simulink model "dq_model"  (R2015a)
settings: Solver=ode45  StartTime=0.0  StopTime=1.5  FixedStep=1e-5  MaxStep=1e-3  RelTol=1e-3
InitFcn:
  | parametriAM
values from neighbouring files (symbols this model uses):
  Imrn = 7.4    [parametriAM.m]
  Ismax = In*sqrt(2)    [parametriAM.m]
  J = 0.019    [parametriAM.m]    (also in podatki.m = 0.01)
  Ki_Imr = 1000    [parametriAM.m]
  Ki_tok = 5.0    (= 5)    [parametriAM.m]
  Ki_wr = 1000    [parametriAM.m]
  Kp_Imr = 100    [parametriAM.m]
  Kp_tok = 0.05    [parametriAM.m]
  Kp_wr = 50    [parametriAM.m]
  Lm = 0.0493    [parametriAM.m]    (also in podatki.m = 0.2342)
  Lr = 0.05315    [parametriAM.m]    (also in podatki.m = 0.2449)
  Ls = 0.05315    [parametriAM.m]    (also in podatki.m = 0.2449)
  Lst = sigma*Ls    (= 0.00742111947319)    [parametriAM.m]
  pp = 3    [parametriAM.m]    (also in podatki.m = 2)
  Rs = 0.594    [parametriAM.m]    (also in podatki.m = 3.7)
  sigma = 1 - 1/((1+sigmaR)*(1+sigmaS))    (= 0.13962595434)    [parametriAM.m]
  Tr = Lr/Rr    (= 0.0771407837446)    [parametriAM.m]
  Udc = Un*sqrt(2)    [parametriAM.m]
  wb_upper_limit_field_weaking = sqrt((Ls^2+Lst^2)/(2*Lst^2*Ls^2))*Usmax/Ismax    [parametriAM.m]
  wn = Udc/sqrt(Ls^2*(Imrn)^2+Lst^2*(Ismax^2-(Imrn)^2))    [maximalnaelipsa.m]    (also in parametriAM.m = Un/sqrt(Ls^2*(Imrn)^2+Lst^2*(Ismax^2-(Imrn)^2))/pp)
libraries: simulink x20
(part 1 of 2)
settings Model: CovModelRefEnable=off  Creator=Mitja1  LastModifiedBy=Jan
settings DataIOCC: LimitDataPoints=off  SaveFormat=Dataset
settings HardwareCC: ProdBitPerPointer=64  ProdLargestAtomicFloat=Float  ProdIntDivRoundTo=Zero  ProdEndianess=LittleEndian  ProdHWDeviceType=Specified
settings ModelReferenceCC: PropagateSignalLabelsOutOfModel=on

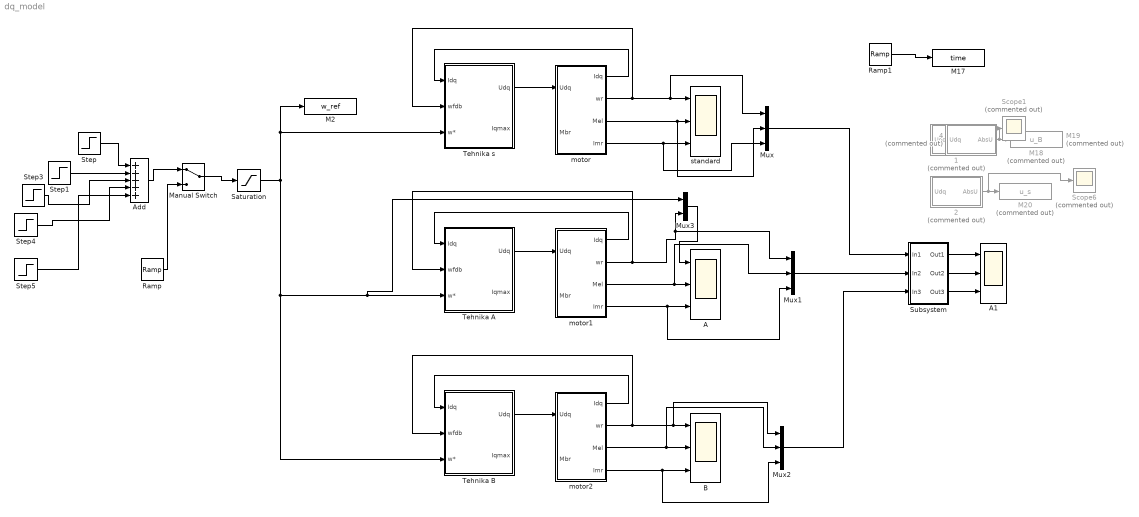
== system dq_model ==
  1 : Subsystem  Commented=on
  2 : Subsystem  Commented=on
  4 : Subsystem  Commented=on
  A : Scope  NumInputPorts=3
      settings: TimeRange=auto  MaxDataPoints=5000  SaveToWorkspace=off  SaveName=ScopeData5  YMin=-48.75~-0.06733~-3.30469  YMax=438.75~0.60598~29.7522  SampleTime=-1
  A1 : Scope  NumInputPorts=3
      settings: TimeRange=auto  MaxDataPoints=5000  SaveToWorkspace=off  SaveName=ScopeData7  YMin=-65.4584~-0.02651~-3.33779  YMax=589.12557~0.12258~30.05009  SampleTime=-1
  Add : Sum  Inputs=+++++
  B : Scope  NumInputPorts=3
      settings: TimeRange=auto  MaxDataPoints=5000  SaveToWorkspace=off  SaveName=ScopeData6  YMin=-28.02182~-2.20302~-3.30355  YMax=252.1964~2.96621~29.74192  SampleTime=-1
  M17 : ToWorkspace  VariableName=time  SampleTime=-1
      settings: Decimation=3  Save2DSignal=2-D array (concatenate along first dimension)
  M18 : ToWorkspace  Commented=on  VariableName=u_A  SampleTime=-1
      settings: Decimation=3  Save2DSignal=2-D array (concatenate along first dimension)
  M19 : ToWorkspace  Commented=on  VariableName=u_B  SampleTime=-1
      settings: Decimation=3  Save2DSignal=2-D array (concatenate along first dimension)
  M2 : ToWorkspace  VariableName=w_ref  SampleTime=-1
      settings: Decimation=3  Save2DSignal=2-D array (concatenate along first dimension)
  M20 : ToWorkspace  Commented=on  VariableName=u_s  SampleTime=-1
      settings: Decimation=3  Save2DSignal=2-D array (concatenate along first dimension)
  Manual Switch : ManualSwitch
  Mux : Mux  Inputs=3
  Mux1 : Mux  Inputs=3
  Mux2 : Mux  Inputs=3
  Mux3 : Mux  Inputs=2
  Ramp : simulink/Sources/Ramp  slope=20  start=0.5  X0=0
  Ramp1 : simulink/Sources/Ramp  slope=1  start=0  X0=0
  Saturation : Saturate  UpperLimit=352.3943*3  LowerLimit=-352.3943*3
  Scope1 : Scope  Commented=on
      settings: TimeRange=auto  MaxDataPoints=5000  SaveToWorkspace=off  YMin=-4.24545  YMax=40.8883  SampleTime=-1
  Scope6 : Scope  Commented=on
      settings: TimeRange=auto  MaxDataPoints=5000  SaveToWorkspace=off  SaveName=ScopeData14  YMin=-2.3666  YMax=41.08778  SampleTime=-1
  Step : Step  Time=0.2  After=1000*2*pi/60  SampleTime=0
  Step1 : Step  Time=0.4  After=1000*2*pi/60  SampleTime=0
  Step3 : Step  Time=0.6  After=1000*2*pi/60  SampleTime=0
  Step4 : Step  Time=0.8  After=1000*2*pi/60  SampleTime=0
  Step5 : Step  After=1000*2*pi/60  SampleTime=0
  Subsystem : Subsystem
  Tehnika A : Subsystem
  Tehnika B : Subsystem
  Tehnika s : Subsystem
  motor : Subsystem
  motor1 : Subsystem
  motor2 : Subsystem
  standard : Scope  NumInputPorts=3
      settings: TimeRange=auto  MaxDataPoints=5000  SaveToWorkspace=off  YMin=-65.46543~-2.0827~-3.30486  YMax=589.18883~3.06396~29.75373  SampleTime=-1
  wires:
  Step/1 -> Add/1
  Add/1 -> Manual Switch/1
  Ramp1/1 -> M17/1
  2/1(AbsU) -> Scope6/1, M20/1
  1/1(AbsU) -> M19/1
  4/1(AbsU) -> Scope1/1, M18/1
  Manual Switch/1 -> Saturation/1
  motor/1(Idq) -> Tehnika s/1(Idq)
  motor/2(wr) -> Tehnika s/2(wfdb), Mux/1, standard/1
  Ramp/1 -> Manual Switch/2
  motor/4(Imr) -> Mux/3, standard/3
  Tehnika s/1(Udq) -> motor/1(Udq)
  motor/3(Mel) -> Mux/2, standard/2
  Step1/1 -> Add/2
  Step3/1 -> Add/3
  Step4/1 -> Add/4
  Step5/1 -> Add/5
  motor1/1(Idq) -> Tehnika A/1(Idq)
  motor1/2(wr) -> Mux1/1, Mux3/2, Tehnika A/2(wfdb)
  motor1/4(Imr) -> Mux1/3, A/3
  Tehnika A/1(Udq) -> motor1/1(Udq)
  motor1/3(Mel) -> Mux1/2, A/2
  motor2/1(Idq) -> Tehnika B/1(Idq)
  motor2/2(wr) -> Tehnika B/2(wfdb), Mux2/1, B/1
  motor2/4(Imr) -> Mux2/3, B/3
  Tehnika B/1(Udq) -> motor2/1(Udq)
  motor2/3(Mel) -> Mux2/2, B/2
  Mux/1 -> Subsystem/1(In1)
  Mux1/1 -> Subsystem/2(In2)
  Mux2/1 -> Subsystem/3(In3)
  Subsystem/2(Out2) -> A1/2
  Subsystem/1(Out1) -> A1/1
  Subsystem/3(Out3) -> A1/3
  Mux3/1 -> A/1
  Saturation/1 -> Tehnika s/3(w*), M2/1, Tehnika B/3(w*), Mux3/1, Tehnika A/3(w*)

== system dq_model/1 ==
  Udq : Inport
  Abs : Abs
  Demux : Demux  Outputs=2
  Real-Imag to Complex : RealImagToComplex
  AbsU : Outport
  wires:
  Abs/1 -> AbsU/1
  Real-Imag to Complex/1 -> Abs/1
  Demux/1 -> Real-Imag to Complex/1
  Demux/2 -> Real-Imag to Complex/2
  Udq/1 -> Demux/1

== system dq_model/2 ==
  Udq : Inport
  Abs : Abs
  Demux : Demux  Outputs=2
  Real-Imag to Complex : RealImagToComplex
  AbsU : Outport
  wires:
  Udq/1 -> Demux/1
  Demux/2 -> Real-Imag to Complex/2
  Demux/1 -> Real-Imag to Complex/1
  Real-Imag to Complex/1 -> Abs/1
  Abs/1 -> AbsU/1

== system dq_model/4 ==
  Udq : Inport
  Abs : Abs
  Demux : Demux  Outputs=2
  Real-Imag to Complex : RealImagToComplex
  AbsU : Outport
  wires:
  Udq/1 -> Demux/1
  Demux/2 -> Real-Imag to Complex/2
  Demux/1 -> Real-Imag to Complex/1
  Real-Imag to Complex/1 -> Abs/1
  Abs/1 -> AbsU/1

== system dq_model/Subsystem ==
  In1 : Inport
  In2 : Inport  Port=2
  In3 : Inport  Port=3
  Demux : Demux  Outputs=3
  Demux1 : Demux  Outputs=3
  Demux2 : Demux  Outputs=3
  Mux4 : Mux  Inputs=3
  Mux5 : Mux  Inputs=3
  Mux6 : Mux  Inputs=3
  Out1 : Outport
  Out2 : Outport  Port=2
  Out3 : Outport  Port=3
  wires:
  Demux1/3 -> Mux6/2
  In1/1 -> Demux/1
  Mux4/1 -> Out1/1
  Demux2/2 -> Mux5/3
  Demux/1 -> Mux4/1
  Demux/2 -> Mux5/1
  In3/1 -> Demux2/1
  Demux1/2 -> Mux5/2
  Demux/3 -> Mux6/1
  In2/1 -> Demux1/1
  Demux2/3 -> Mux6/3
  Demux2/1 -> Mux4/3
  Mux5/1 -> Out2/1
  Demux1/1 -> Mux4/2
  Mux6/1 -> Out3/1

== system dq_model/Tehnika A ==
  Idq : Inport
  wfdb : Inport  Port=2
  w* : Inport  Port=3
  Gain2 : Gain  Gain=Udc
  M9 : ToWorkspace  VariableName=I_mr_Aref  SampleTime=-1
      settings: Decimation=3  Save2DSignal=2-D array (concatenate along first dimension)
  Magnetilnireg : Subsystem
  Regulacija navora : Subsystem
  TechniqueA1 : Subsystem
  Tok regulator : Subsystem
  Udq : Outport
  Iqmax : Outport  Port=2
  wires:
  Gain2/1 -> Udq/1
  Tok regulator/1(Udq*) -> Gain2/1
  w*/1 -> TechniqueA1/1(wmr), Regulacija navora/1(w*)
  Idq/1 -> Magnetilnireg/1(Idqdej), Regulacija navora/2(Idqdej), Tok regulator/1(Idqdej)
  TechniqueA1/1(6.1-126) -> Magnetilnireg/2(Imr*), M9/1
  Regulacija navora/2(Iqmax) -> Iqmax/1
  Regulacija navora/1(iq*) -> Tok regulator/3(Iq)
  wfdb/1 -> Regulacija navora/3(wfdb)
  Magnetilnireg/1(Id*) -> Tok regulator/2(Id)

== system dq_model/Tehnika B ==
  Idq : Inport
  wfdb : Inport  Port=2
  w* : Inport  Port=3
  Gain2 : Gain  Gain=Udc
  M9 : ToWorkspace  VariableName=I_mr_Bref  SampleTime=-1
      settings: Decimation=3  Save2DSignal=2-D array (concatenate along first dimension)
  Magnetilnireg : Subsystem
  Regulacija navora : Subsystem
  TechniqueB1 : Subsystem
  Tok regulator : Subsystem
  Udq : Outport
  Iqmax : Outport  Port=2
  wires:
  wfdb/1 -> Regulacija navora/3(wfdb)
  Regulacija navora/1(iq*) -> Tok regulator/3(Iq)
  Regulacija navora/2(Iqmax) -> Iqmax/1
  TechniqueB1/1(6.1-135) -> M9/1, Magnetilnireg/2(Imr*)
  Idq/1 -> Tok regulator/1(Idqdej), TechniqueB1/1(Isdq), Regulacija navora/2(Idqdej), Magnetilnireg/1(Idqdej)
  w*/1 -> TechniqueB1/2(w), Regulacija navora/1(w*)
  Tok regulator/1(Udq*) -> Gain2/1
  Gain2/1 -> Udq/1
  Magnetilnireg/1(Id*) -> Tok regulator/2(Id)

== system dq_model/Tehnika s ==
  Idq : Inport
  wfdb : Inport  Port=2
  w* : Inport  Port=3
  Gain2 : Gain  Gain=Udc
  M9 : ToWorkspace  VariableName=I_mr_sref  SampleTime=-1
      settings: Decimation=3  Save2DSignal=2-D array (concatenate along first dimension)
  Magnetilnireg : Subsystem
  Regulacija navora : Subsystem
  TechniqueA2 : Subsystem
  Tok regulator : Subsystem
  Udq : Outport
  Iqmax : Outport  Port=2
  wires:
  wfdb/1 -> TechniqueA2/1(wmr), Regulacija navora/3(wfdb)
  Regulacija navora/1(iq*) -> Tok regulator/3(Iq)
  Regulacija navora/2(Iqmax) -> Iqmax/1
  TechniqueA2/1(Nemec) -> M9/1, Magnetilnireg/2(Imr*)
  Idq/1 -> Tok regulator/1(Idqdej), Regulacija navora/2(Idqdej), Magnetilnireg/1(Idqdej)
  w*/1 -> Regulacija navora/1(w*)
  Tok regulator/1(Udq*) -> Gain2/1
  Gain2/1 -> Udq/1
  Magnetilnireg/1(Id*) -> Tok regulator/2(Id)

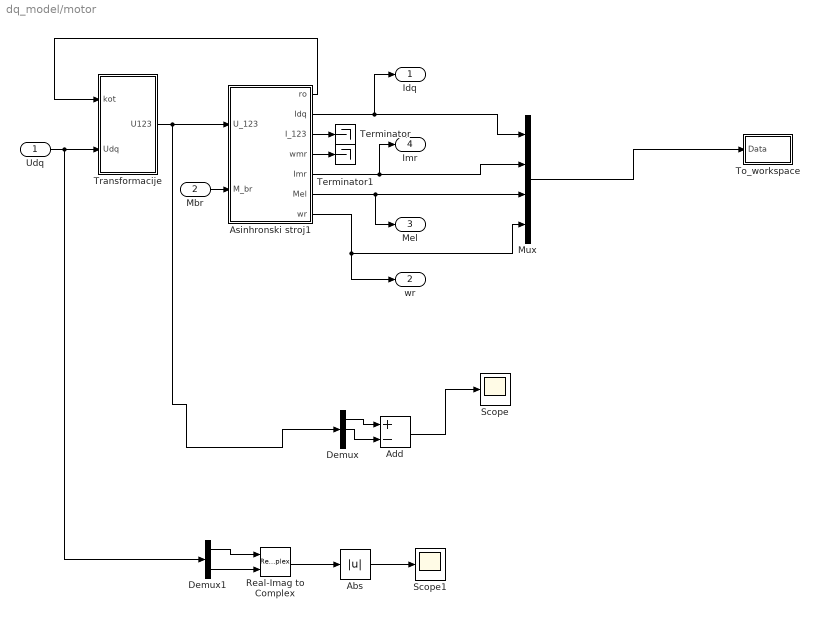
== system dq_model/motor ==
  Udq : Inport
  Mbr : Inport  Port=2
  Abs : Abs
  Add : Sum  Inputs=+-
  Asinhronski stroj1 : Subsystem  InitFcn=parametriAM
  Demux : Demux  Outputs=3
  Demux1 : Demux  Outputs=2
  Mux : Mux
  Real-Imag to Complex : RealImagToComplex
  Scope : Scope
      settings: TimeRange=auto  MaxDataPoints=5000  SaveToWorkspace=off  SaveName=ScopeData3  YMin=-37.49992  YMax=37.49999  SampleTime=-1
  Scope1 : Scope
      settings: TimeRange=auto  MaxDataPoints=5000  SaveToWorkspace=off  YMin=-2.12297  YMax=19.4809  SampleTime=-1
  Terminator : Terminator
  Terminator1 : Terminator
  To_workspace : Subsystem
  Transformacije : Subsystem
  Idq : Outport
  wr : Outport  Port=2
  Mel : Outport  Port=3
  Imr : Outport  Port=4
  wires:
  Mbr/1 -> Asinhronski stroj1/2(M_br)
  Asinhronski stroj1/6(Mel) -> Mux/3, Mel/1
  Asinhronski stroj1/7(wr) -> wr/1, Mux/4
  Asinhronski stroj1/5(Imr) -> Mux/2, Imr/1
  Udq/1 -> Demux1/1, Transformacije/2(Udq)
  Transformacije/1(U123) -> Demux/1, Asinhronski stroj1/1(U_123)
  Asinhronski stroj1/1(ro) -> Transformacije/1(kot)
  Asinhronski stroj1/2(Idq) -> Idq/1, Mux/1
  Mux/1 -> To_workspace/1(Data)
  Asinhronski stroj1/4(wmr) -> Terminator1/1
  Asinhronski stroj1/3(I_123) -> Terminator/1
  Add/1 -> Scope/1
  Demux/1 -> Add/1
  Demux/2 -> Add/2
  Demux1/1 -> Real-Imag to Complex/1
  Demux1/2 -> Real-Imag to Complex/2
  Real-Imag to Complex/1 -> Abs/1
  Abs/1 -> Scope1/1

== system dq_model/motor1 ==
  Udq : Inport
  Mbr : Inport  Port=2
  Asinhronski stroj1 : Subsystem  InitFcn=parametriAM
  Mux : Mux
  Scope : Scope
      settings: TimeRange=auto  MaxDataPoints=5000  SaveToWorkspace=off  SaveName=ScopeData3  YMin=-26.51646  YMax=26.51646  SampleTime=-1
  Terminator : Terminator
  Terminator1 : Terminator
  To_workspace : Subsystem
  Transformacije : Subsystem
  Idq : Outport
  wr : Outport  Port=2
  Mel : Outport  Port=3
  Imr : Outport  Port=4
  wires:
  Asinhronski stroj1/3(I_123) -> Terminator/1
  Asinhronski stroj1/4(wmr) -> Terminator1/1
  Mux/1 -> To_workspace/1(Data)
  Asinhronski stroj1/2(Idq) -> Mux/1, Idq/1
  Asinhronski stroj1/1(ro) -> Transformacije/1(kot)
  Transformacije/1(U123) -> Asinhronski stroj1/1(U_123), Scope/1
  Udq/1 -> Transformacije/2(Udq)
  Asinhronski stroj1/5(Imr) -> Imr/1, Mux/2
  Asinhronski stroj1/7(wr) -> Mux/4, wr/1
  Asinhronski stroj1/6(Mel) -> Mel/1, Mux/3
  Mbr/1 -> Asinhronski stroj1/2(M_br)

== system dq_model/motor2 ==
  Udq : Inport
  Mbr : Inport  Port=2
  Asinhronski stroj1 : Subsystem  InitFcn=parametriAM
  Mux : Mux
  Scope : Scope
      settings: TimeRange=auto  MaxDataPoints=5000  SaveToWorkspace=off  SaveName=ScopeData3  YMin=-26.51646  YMax=26.51646  SampleTime=-1
  Terminator : Terminator
  Terminator1 : Terminator
  To_workspace : Subsystem
  Transformacije : Subsystem
  Idq : Outport
  wr : Outport  Port=2
  Mel : Outport  Port=3
  Imr : Outport  Port=4
  wires:
  Mbr/1 -> Asinhronski stroj1/2(M_br)
  Asinhronski stroj1/6(Mel) -> Mux/3, Mel/1
  Asinhronski stroj1/7(wr) -> wr/1, Mux/4
  Asinhronski stroj1/5(Imr) -> Mux/2, Imr/1
  Udq/1 -> Transformacije/2(Udq)
  Transformacije/1(U123) -> Scope/1, Asinhronski stroj1/1(U_123)
  Asinhronski stroj1/1(ro) -> Transformacije/1(kot)
  Asinhronski stroj1/2(Idq) -> Idq/1, Mux/1
  Mux/1 -> To_workspace/1(Data)
  Asinhronski stroj1/4(wmr) -> Terminator1/1
  Asinhronski stroj1/3(I_123) -> Terminator/1

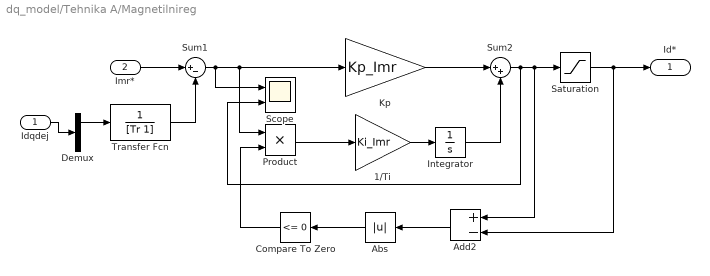
== system dq_model/Tehnika A/Magnetilnireg ==
  Idqdej : Inport
  Imr* : Inport  Port=2
  1/Ti : Gain  Gain=Ki_Imr  SaturateOnIntegerOverflow=on  OutDataTypeStr=Inherit: Same as input  ParamDataTypeStr=Inherit: Same as input
  Abs : Abs  ZeroCross=off
  Add2 : Sum  Inputs=+-
  Compare To Zero : simulink/Logic and Bit Operations/Compare To Zero  relop=<=  OutDataTypeStr=boolean  ZeroCross=off
  Demux : Demux  Outputs=2
  Integrator : Integrator
  Kp : Gain  Gain=Kp_Imr  SaturateOnIntegerOverflow=on  OutDataTypeStr=Inherit: Same as input  ParamDataTypeStr=Inherit: Same as input
  Product : Product
  Saturation : Saturate  UpperLimit=Ismax  LowerLimit=-Ismax  ZeroCross=off
  Scope : Scope  NumInputPorts=2
      settings: TimeRange=auto  MaxDataPoints=5000  SaveToWorkspace=off  SaveName=ScopeData6  YMin=-0.95903~-5  YMax=1.63998~5  SampleTime=-1
  Sum1 : Sum  Inputs=|+-
  Sum2 : Sum  Inputs=|++
  Transfer Fcn : TransferFcn  Denominator=[Tr 1]
  Id* : Outport
  wires:
  Sum1/1 -> Scope/1, Product/1, Kp/1
  Add2/1 -> Abs/1
  Abs/1 -> Compare To Zero/1
  1/Ti/1 -> Integrator/1
  Product/1 -> 1/Ti/1
  Kp/1 -> Sum2/1
  Compare To Zero/1 -> Product/2
  Sum2/1 -> Scope/2, Add2/1, Saturation/1
  Integrator/1 -> Sum2/2
  Imr*/1 -> Sum1/1
  Saturation/1 -> Add2/2, Id*/1
  Demux/1 -> Transfer Fcn/1
  Transfer Fcn/1 -> Sum1/2
  Idqdej/1 -> Demux/1

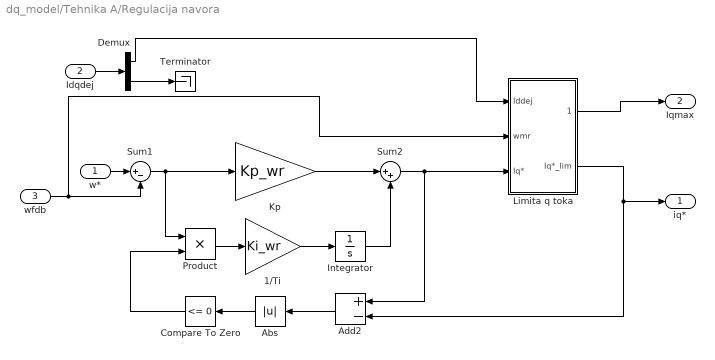
== system dq_model/Tehnika A/Regulacija navora ==
  w* : Inport
  Idqdej : Inport  Port=2
  wfdb : Inport  Port=3
  1/Ti : Gain  Gain=Ki_wr  SaturateOnIntegerOverflow=on  OutDataTypeStr=Inherit: Same as input  ParamDataTypeStr=Inherit: Same as input
  Abs : Abs  ZeroCross=off
  Add2 : Sum  Inputs=+-
  Compare To Zero : simulink/Logic and Bit Operations/Compare To Zero  relop=<=  OutDataTypeStr=boolean  ZeroCross=off
  Demux : Demux  Outputs=2
  Integrator : Integrator
  Kp : Gain  Gain=Kp_wr  SaturateOnIntegerOverflow=on  OutDataTypeStr=Inherit: Same as input  ParamDataTypeStr=Inherit: Same as input
  Limita q toka : Subsystem
  Product : Product
  Sum1 : Sum  Inputs=|+-
  Sum2 : Sum  Inputs=|++
  Terminator : Terminator
  iq* : Outport
  Iqmax : Outport  Port=2
  wires:
  1/Ti/1 -> Integrator/1
  Sum1/1 -> Product/1, Kp/1
  Integrator/1 -> Sum2/2
  Add2/1 -> Abs/1
  Abs/1 -> Compare To Zero/1
  Kp/1 -> Sum2/1
  Compare To Zero/1 -> Product/2
  Product/1 -> 1/Ti/1
  w*/1 -> Sum1/1
  Limita q toka/2(Iq*_lim) -> iq*/1, Add2/2
  Idqdej/1 -> Demux/1
  Limita q toka/1(Iqmaxlim) -> Iqmax/1
  Demux/1 -> Limita q toka/1(Iddej)
  Sum2/1 -> Limita q toka/3(Iq*), Add2/1
  wfdb/1 -> Limita q toka/2(wmr), Sum1/2
  Demux/2 -> Terminator/1

== system dq_model/Tehnika A/TechniqueA1 ==
  wmr : Inport
  Abs : Abs
  Add : Sum
  Add1 : Sum  Inputs=+-
  Constant1 : Constant  Value=0.000001
  Constant3 : Constant  Value=Udc
  Constant4 : Constant  Value=Lst^2*Ismax^2
  Divide1 : Product  Inputs=*/
  Gain : Gain  Gain=1/(Ls^2-Lst^2)
  Gain1 : Gain
  Gain2 : Gain  Gain=pp
  Product1 : Product
  Saturation1 : Saturate  UpperLimit=+Imrn*sqrt(2)  LowerLimit=0
  Signed Sqrt : Sqrt  Operator=signedSqrt  OutputSignalType=real  SaturateOnIntegerOverflow=on
  6.1-126 : Outport
  wires:
  Add/1 -> Divide1/2
  Abs/1 -> Add/1
  Constant1/1 -> Add/2
  Constant3/1 -> Divide1/1
  Divide1/1 -> Product1/2, Product1/1
  Product1/1 -> Add1/1
  Saturation1/1 -> 6.1-126/1
  Add1/1 -> Gain/1
  Gain/1 -> Signed Sqrt/1
  Signed Sqrt/1 -> Saturation1/1
  Gain2/1 -> Abs/1
  Constant4/1 -> Gain1/1
  Gain1/1 -> Add1/2
  wmr/1 -> Gain2/1

== system dq_model/Tehnika A/Tok regulator ==
  Idqdej : Inport
  Id : Inport  Port=2
  Iq : Inport  Port=3
  Demux : Demux  Outputs=2
  Dregulator : Subsystem
  Limita Uq : Subsystem
  Mux : Mux  Inputs=2
  Qregulator : Subsystem
  Scope : Scope  NumInputPorts=2
      settings: TimeRange=auto  MaxDataPoints=5000  SaveToWorkspace=off  SaveName=ScopeData11  YMin=-4.07237~-5  YMax=36.65013~5  SampleTime=-1
  Udq* : Outport
  wires:
  Mux/1 -> Udq*/1
  Idqdej/1 -> Demux/1
  Limita Uq/1(Uq_lim) -> Qregulator/3(Uqlim), Mux/2
  Dregulator/1(Ud*(-1:1)) -> Mux/1, Limita Uq/1(Ud)
  Id/1 -> Dregulator/1(Id*)
  Demux/1 -> Dregulator/2(Iddej)
  Iq/1 -> Scope/2, Qregulator/2(Iq*)
  Demux/2 -> Scope/1, Qregulator/1(Iqdej)
  Qregulator/1(Uq*(-1:1)) -> Limita Uq/2(Uq)

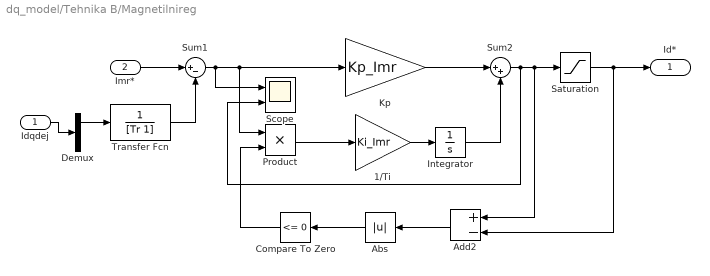
== system dq_model/Tehnika B/Magnetilnireg ==
  Idqdej : Inport
  Imr* : Inport  Port=2
  1/Ti : Gain  Gain=Ki_Imr  SaturateOnIntegerOverflow=on  OutDataTypeStr=Inherit: Same as input  ParamDataTypeStr=Inherit: Same as input
  Abs : Abs  ZeroCross=off
  Add2 : Sum  Inputs=+-
  Compare To Zero : simulink/Logic and Bit Operations/Compare To Zero  relop=<=  OutDataTypeStr=boolean  ZeroCross=off
  Demux : Demux  Outputs=2
  Integrator : Integrator
  Kp : Gain  Gain=Kp_Imr  SaturateOnIntegerOverflow=on  OutDataTypeStr=Inherit: Same as input  ParamDataTypeStr=Inherit: Same as input
  Product : Product
  Saturation : Saturate  UpperLimit=Ismax  LowerLimit=-Ismax  ZeroCross=off
  Scope : Scope  NumInputPorts=2
      settings: TimeRange=auto  MaxDataPoints=5000  SaveToWorkspace=off  SaveName=ScopeData6  YMin=-0.95903~-5  YMax=1.63998~5  SampleTime=-1
  Sum1 : Sum  Inputs=|+-
  Sum2 : Sum  Inputs=|++
  Transfer Fcn : TransferFcn  Denominator=[Tr 1]
  Id* : Outport
  wires:
  Idqdej/1 -> Demux/1
  Transfer Fcn/1 -> Sum1/2
  Demux/1 -> Transfer Fcn/1
  Saturation/1 -> Id*/1, Add2/2
  Imr*/1 -> Sum1/1
  Integrator/1 -> Sum2/2
  Sum2/1 -> Saturation/1, Add2/1, Scope/2
  Compare To Zero/1 -> Product/2
  Kp/1 -> Sum2/1
  Product/1 -> 1/Ti/1
  1/Ti/1 -> Integrator/1
  Abs/1 -> Compare To Zero/1
  Add2/1 -> Abs/1
  Sum1/1 -> Kp/1, Product/1, Scope/1

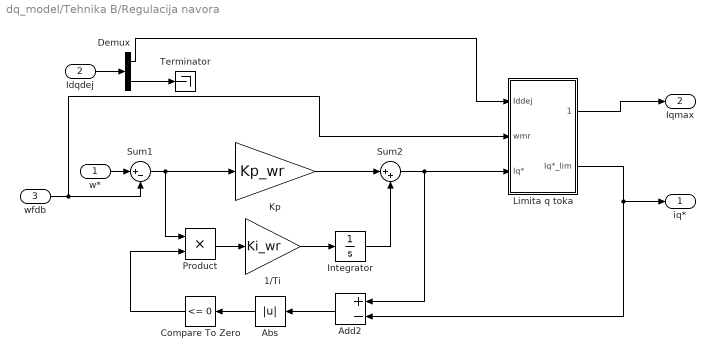
== system dq_model/Tehnika B/Regulacija navora ==
  w* : Inport
  Idqdej : Inport  Port=2
  wfdb : Inport  Port=3
  1/Ti : Gain  Gain=Ki_wr  SaturateOnIntegerOverflow=on  OutDataTypeStr=Inherit: Same as input  ParamDataTypeStr=Inherit: Same as input
  Abs : Abs  ZeroCross=off
  Add2 : Sum  Inputs=+-
  Compare To Zero : simulink/Logic and Bit Operations/Compare To Zero  relop=<=  OutDataTypeStr=boolean  ZeroCross=off
  Demux : Demux  Outputs=2
  Integrator : Integrator
  Kp : Gain  Gain=Kp_wr  SaturateOnIntegerOverflow=on  OutDataTypeStr=Inherit: Same as input  ParamDataTypeStr=Inherit: Same as input
  Limita q toka : Subsystem
  Product : Product
  Sum1 : Sum  Inputs=|+-
  Sum2 : Sum  Inputs=|++
  Terminator : Terminator
  iq* : Outport
  Iqmax : Outport  Port=2
  wires:
  Demux/2 -> Terminator/1
  wfdb/1 -> Sum1/2, Limita q toka/2(wmr)
  Sum2/1 -> Add2/1, Limita q toka/3(Iq*)
  Demux/1 -> Limita q toka/1(Iddej)
  Limita q toka/1(Iqmaxlim) -> Iqmax/1
  Idqdej/1 -> Demux/1
  Limita q toka/2(Iq*_lim) -> Add2/2, iq*/1
  w*/1 -> Sum1/1
  Product/1 -> 1/Ti/1
  Compare To Zero/1 -> Product/2
  Kp/1 -> Sum2/1
  Abs/1 -> Compare To Zero/1
  Add2/1 -> Abs/1
  Integrator/1 -> Sum2/2
  Sum1/1 -> Kp/1, Product/1
  1/Ti/1 -> Integrator/1

== system dq_model/Tehnika B/TechniqueB1 ==
  Isdq : Inport
  w : Inport  Port=2
  Add4 : Sum
  Const c : Subsystem
  Deljeno imenovalec 6.1-135 : Gain  Gain=1/(Ls^2-Lst^2)
  Demux : Demux  Outputs=2
  Gain4 : Gain  Gain=-Ls
  Gain6 : Gain  Gain=pp
  Korenski del : Subsystem
  Saturation : Saturate  UpperLimit=+Imrn*sqrt(2)  LowerLimit=-Imrn*sqrt(2)
  Scope : Scope
      settings: TimeRange=auto  MaxDataPoints=5000  SaveToWorkspace=off  SaveName=ScopeData5  YMin=-0.09404  YMax=0.14273  SampleTime=-1
  Terminator : Terminator
  6.1-135 : Outport
  wires:
  Demux/1 -> Const c/1(Id)
  Demux/2 -> Terminator/1
  Saturation/1 -> 6.1-135/1
  Const c/1(c) -> Scope/1, Korenski del/1(c), Gain4/1
  Gain4/1 -> Add4/1
  Add4/1 -> Deljeno imenovalec 6.1-135/1
  Deljeno imenovalec 6.1-135/1 -> Saturation/1
  Isdq/1 -> Demux/1
  Korenski del/1(korenjen del) -> Add4/2
  w/1 -> Gain6/1
  Gain6/1 -> Korenski del/2(w)

== system dq_model/Tehnika B/Tok regulator ==
  Idqdej : Inport
  Id : Inport  Port=2
  Iq : Inport  Port=3
  Demux : Demux  Outputs=2
  Dregulator : Subsystem
  Limita Uq : Subsystem
  Mux : Mux  Inputs=2
  Qregulator : Subsystem
  Scope : Scope  NumInputPorts=2
      settings: TimeRange=auto  MaxDataPoints=5000  SaveToWorkspace=off  SaveName=ScopeData11  YMin=-4.07237~-5  YMax=36.65013~5  SampleTime=-1
  Udq* : Outport
  wires:
  Qregulator/1(Uq*(-1:1)) -> Limita Uq/2(Uq)
  Demux/2 -> Qregulator/1(Iqdej), Scope/1
  Iq/1 -> Qregulator/2(Iq*), Scope/2
  Demux/1 -> Dregulator/2(Iddej)
  Id/1 -> Dregulator/1(Id*)
  Dregulator/1(Ud*(-1:1)) -> Limita Uq/1(Ud), Mux/1
  Limita Uq/1(Uq_lim) -> Mux/2, Qregulator/3(Uqlim)
  Idqdej/1 -> Demux/1
  Mux/1 -> Udq*/1

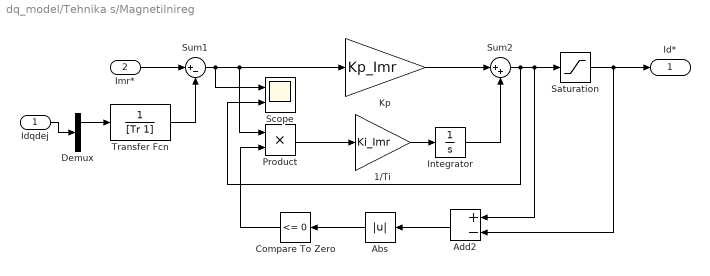
== system dq_model/Tehnika s/Magnetilnireg ==
  Idqdej : Inport
  Imr* : Inport  Port=2
  1/Ti : Gain  Gain=Ki_Imr  SaturateOnIntegerOverflow=on  OutDataTypeStr=Inherit: Same as input  ParamDataTypeStr=Inherit: Same as input
  Abs : Abs  ZeroCross=off
  Add2 : Sum  Inputs=+-
  Compare To Zero : simulink/Logic and Bit Operations/Compare To Zero  relop=<=  OutDataTypeStr=boolean  ZeroCross=off
  Demux : Demux  Outputs=2
  Integrator : Integrator
  Kp : Gain  Gain=Kp_Imr  SaturateOnIntegerOverflow=on  OutDataTypeStr=Inherit: Same as input  ParamDataTypeStr=Inherit: Same as input
  Product : Product
  Saturation : Saturate  UpperLimit=Ismax  LowerLimit=-Ismax  ZeroCross=off
  Scope : Scope  NumInputPorts=2
      settings: TimeRange=auto  MaxDataPoints=5000  SaveToWorkspace=off  SaveName=ScopeData6  YMin=-0.95903~-5  YMax=1.63998~5  SampleTime=-1
  Sum1 : Sum  Inputs=|+-
  Sum2 : Sum  Inputs=|++
  Transfer Fcn : TransferFcn  Denominator=[Tr 1]
  Id* : Outport
  wires:
  Idqdej/1 -> Demux/1
  Transfer Fcn/1 -> Sum1/2
  Demux/1 -> Transfer Fcn/1
  Saturation/1 -> Id*/1, Add2/2
  Imr*/1 -> Sum1/1
  Integrator/1 -> Sum2/2
  Sum2/1 -> Saturation/1, Add2/1, Scope/2
  Compare To Zero/1 -> Product/2
  Kp/1 -> Sum2/1
  Product/1 -> 1/Ti/1
  1/Ti/1 -> Integrator/1
  Abs/1 -> Compare To Zero/1
  Add2/1 -> Abs/1
  Sum1/1 -> Kp/1, Product/1, Scope/1

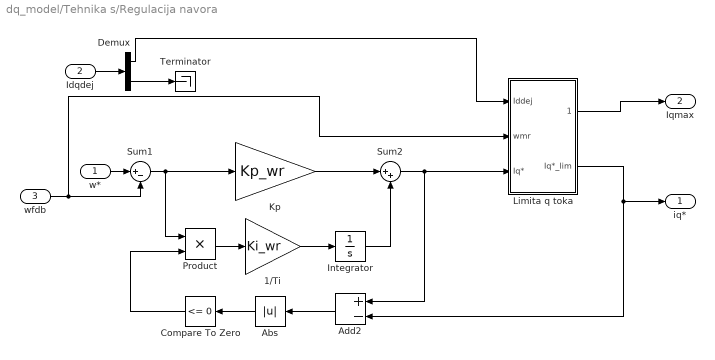
== system dq_model/Tehnika s/Regulacija navora ==
  w* : Inport
  Idqdej : Inport  Port=2
  wfdb : Inport  Port=3
  1/Ti : Gain  Gain=Ki_wr  SaturateOnIntegerOverflow=on  OutDataTypeStr=Inherit: Same as input  ParamDataTypeStr=Inherit: Same as input
  Abs : Abs
  Add2 : Sum  Inputs=+-
  Compare To Zero : simulink/Logic and Bit Operations/Compare To Zero  relop=<=  OutDataTypeStr=boolean
  Demux : Demux  Outputs=2
  Integrator : Integrator
  Kp : Gain  Gain=Kp_wr  SaturateOnIntegerOverflow=on  OutDataTypeStr=Inherit: Same as input  ParamDataTypeStr=Inherit: Same as input
  Limita q toka : Subsystem
  Product : Product
  Sum1 : Sum  Inputs=|+-
  Sum2 : Sum  Inputs=|++
  Terminator : Terminator
  iq* : Outport
  Iqmax : Outport  Port=2
  wires:
  Demux/2 -> Terminator/1
  wfdb/1 -> Sum1/2, Limita q toka/2(wmr)
  Sum2/1 -> Add2/1, Limita q toka/3(Iq*)
  Demux/1 -> Limita q toka/1(Iddej)
  Limita q toka/1(Iqmaxlim) -> Iqmax/1
  Idqdej/1 -> Demux/1
  Limita q toka/2(Iq*_lim) -> Add2/2, iq*/1
  w*/1 -> Sum1/1
  Product/1 -> 1/Ti/1
  Compare To Zero/1 -> Product/2
  Kp/1 -> Sum2/1
  Abs/1 -> Compare To Zero/1
  Add2/1 -> Abs/1
  Integrator/1 -> Sum2/2
  Sum1/1 -> Kp/1, Product/1
  1/Ti/1 -> Integrator/1

== system dq_model/Tehnika s/TechniqueA2 ==
  wmr : Inport
  Abs : Abs
  Add : Sum
  Constant : Constant  Value=wn*0.9
  Constant1 : Constant  Value=0.000001
  Constant2 : Constant  Value=Imrn*sqrt(2)
  Divide : Product  Inputs=*/
  Product : Product
  Saturation : Saturate  UpperLimit=+Imrn*sqrt(2)  LowerLimit=-Imrn*sqrt(2)
  Nemec : Outport
  wires:
  wmr/1 -> Abs/1
  Saturation/1 -> Nemec/1
  Constant1/1 -> Add/2
  Abs/1 -> Add/1
  Add/1 -> Divide/2
  Constant/1 -> Divide/1
  Product/1 -> Saturation/1
  Divide/1 -> Product/2
  Constant2/1 -> Product/1

== system dq_model/Tehnika s/Tok regulator ==
  Idqdej : Inport
  Id : Inport  Port=2
  Iq : Inport  Port=3
  Demux : Demux  Outputs=2
  Dregulator : Subsystem
  Limita Uq : Subsystem
  Mux : Mux  Inputs=2
  Qregulator : Subsystem
  Scope : Scope  NumInputPorts=2
      settings: TimeRange=auto  MaxDataPoints=5000  SaveToWorkspace=off  SaveName=ScopeData11  YMin=-4.99397~-5  YMax=44.94575~5  SampleTime=-1
  Udq* : Outport
  wires:
  Qregulator/1(Uq*(-1:1)) -> Limita Uq/2(Uq)
  Demux/2 -> Qregulator/1(Iqdej), Scope/1
  Iq/1 -> Qregulator/2(Iq*), Scope/2
  Demux/1 -> Dregulator/2(Iddej)
  Id/1 -> Dregulator/1(Id*)
  Dregulator/1(Ud*(-1:1)) -> Limita Uq/1(Ud), Mux/1
  Limita Uq/1(Uq_lim) -> Mux/2, Qregulator/3(Uqlim)
  Idqdej/1 -> Demux/1
  Mux/1 -> Udq*/1

== system dq_model/motor/Asinhronski stroj1 ==
  U_123 : Inport
  M_br : Inport  Port=2
  Clarke : Subsystem
  Inverzni Clarke : Subsystem
  Inverzni Park : Subsystem
  Mehanika : Subsystem
  Park : Subsystem
  napetostni dq model : Subsystem
  ro : Outport
  Idq : Outport  Port=2
  I_123 : Outport  Port=3
  wmr : Outport  Port=4
  Imr : Outport  Port=5
  Mel : Outport  Port=6
  wr : Outport  Port=7
  wires:
  Inverzni Park/1(I_ab) -> Inverzni Clarke/1(I_ab)
  Clarke/1(U_ab) -> Park/1(U_ab)
  Mehanika/1(wr) -> napetostni dq model/2(wr), wr/1
  M_br/1 -> Mehanika/1(M_br)
  napetostni dq model/1(Mel) -> Mel/1, Mehanika/2(M_el)
  Inverzni Clarke/1(I_123) -> I_123/1
  napetostni dq model/4(wmr) -> wmr/1
  napetostni dq model/3(Imr) -> Imr/1
  U_123/1 -> Clarke/1(U_123)
  napetostni dq model/2(Is_dq) -> Idq/1, Inverzni Park/1(I_dq)
  napetostni dq model/5(ro) -> ro/1, Park/2(kot), Inverzni Park/2(kot)
  Park/1(U_dq) -> napetostni dq model/1(Us_dq)

== system dq_model/motor/To_workspace ==
  Data : Inport
  Demux : Demux
  M1 : ToWorkspace  VariableName=Idq_s  SampleTime=-1
      settings: Decimation=3  Save2DSignal=2-D array (concatenate along first dimension)
  M10 : ToWorkspace  VariableName=w_fdb_s  SampleTime=-1
      settings: Decimation=3  Save2DSignal=2-D array (concatenate along first dimension)
  M5 : ToWorkspace  VariableName=M_el_s  SampleTime=-1
      settings: Decimation=3  Save2DSignal=2-D array (concatenate along first dimension)
  M9 : ToWorkspace  VariableName=I_mr_s  SampleTime=-1
      settings: Decimation=3  Save2DSignal=2-D array (concatenate along first dimension)
  wires:
  Demux/4 -> M10/1
  Data/1 -> Demux/1
  Demux/1 -> M1/1
  Demux/2 -> M9/1
  Demux/3 -> M5/1

== system dq_model/motor/Transformacije ==
  kot : Inport
  Udq : Inport  Port=2
  Inverzni Clarke : Subsystem
  Inverzni Park : Subsystem
  U123 : Outport
  wires:
  Inverzni Clarke/1(U_123) -> U123/1
  kot/1 -> Inverzni Park/1(kot)
  Inverzni Park/1(U_ab) -> Inverzni Clarke/1(U_ab)
  Udq/1 -> Inverzni Park/2(U_dq)

== system dq_model/motor1/Asinhronski stroj1 ==
  U_123 : Inport
  M_br : Inport  Port=2
  Clarke : Subsystem
  Inverzni Clarke : Subsystem
  Inverzni Park : Subsystem
  Mehanika : Subsystem
  Park : Subsystem
  napetostni dq model : Subsystem
  ro : Outport
  Idq : Outport  Port=2
  I_123 : Outport  Port=3
  wmr : Outport  Port=4
  Imr : Outport  Port=5
  Mel : Outport  Port=6
  wr : Outport  Port=7
  wires:
  Park/1(U_dq) -> napetostni dq model/1(Us_dq)
  napetostni dq model/5(ro) -> Inverzni Park/2(kot), Park/2(kot), ro/1
  napetostni dq model/2(Is_dq) -> Inverzni Park/1(I_dq), Idq/1
  U_123/1 -> Clarke/1(U_123)
  napetostni dq model/3(Imr) -> Imr/1
  napetostni dq model/4(wmr) -> wmr/1
  Inverzni Clarke/1(I_123) -> I_123/1
  napetostni dq model/1(Mel) -> Mehanika/2(M_el), Mel/1
  M_br/1 -> Mehanika/1(M_br)
  Mehanika/1(wr) -> wr/1, napetostni dq model/2(wr)
  Clarke/1(U_ab) -> Park/1(U_ab)
  Inverzni Park/1(I_ab) -> Inverzni Clarke/1(I_ab)

== system dq_model/motor1/To_workspace ==
  Data : Inport
  Demux : Demux
  M1 : ToWorkspace  VariableName=Idq_A  SampleTime=-1
      settings: Decimation=3  Save2DSignal=2-D array (concatenate along first dimension)
  M10 : ToWorkspace  VariableName=w_fdb_A  SampleTime=-1
      settings: Decimation=3  Save2DSignal=2-D array (concatenate along first dimension)
  M5 : ToWorkspace  VariableName=M_el_A  SampleTime=-1
      settings: Decimation=3  Save2DSignal=2-D array (concatenate along first dimension)
  M9 : ToWorkspace  VariableName=I_mr_A  SampleTime=-1
      settings: Decimation=3  Save2DSignal=2-D array (concatenate along first dimension)
  wires:
  Demux/3 -> M5/1
  Demux/2 -> M9/1
  Demux/1 -> M1/1
  Data/1 -> Demux/1
  Demux/4 -> M10/1

== system dq_model/motor1/Transformacije ==
  kot : Inport
  Udq : Inport  Port=2
  Inverzni Clarke : Subsystem
  Inverzni Park : Subsystem
  U123 : Outport
  wires:
  Udq/1 -> Inverzni Park/2(U_dq)
  Inverzni Park/1(U_ab) -> Inverzni Clarke/1(U_ab)
  kot/1 -> Inverzni Park/1(kot)
  Inverzni Clarke/1(U_123) -> U123/1

== system dq_model/motor2/Asinhronski stroj1 ==
  U_123 : Inport
  M_br : Inport  Port=2
  Clarke : Subsystem
  Inverzni Clarke : Subsystem
  Inverzni Park : Subsystem
  Mehanika : Subsystem
  Park : Subsystem
  napetostni dq model : Subsystem
  ro : Outport
  Idq : Outport  Port=2
  I_123 : Outport  Port=3
  wmr : Outport  Port=4
  Imr : Outport  Port=5
  Mel : Outport  Port=6
  wr : Outport  Port=7
  wires:
  Inverzni Park/1(I_ab) -> Inverzni Clarke/1(I_ab)
  Clarke/1(U_ab) -> Park/1(U_ab)
  Mehanika/1(wr) -> napetostni dq model/2(wr), wr/1
  M_br/1 -> Mehanika/1(M_br)
  napetostni dq model/1(Mel) -> Mel/1, Mehanika/2(M_el)
  Inverzni Clarke/1(I_123) -> I_123/1
  napetostni dq model/4(wmr) -> wmr/1
  napetostni dq model/3(Imr) -> Imr/1
  U_123/1 -> Clarke/1(U_123)
  napetostni dq model/2(Is_dq) -> Idq/1, Inverzni Park/1(I_dq)
  napetostni dq model/5(ro) -> ro/1, Park/2(kot), Inverzni Park/2(kot)
  Park/1(U_dq) -> napetostni dq model/1(Us_dq)

== system dq_model/motor2/To_workspace ==
  Data : Inport
  Demux : Demux
  M1 : ToWorkspace  VariableName=Idq_B  SampleTime=-1
      settings: Decimation=3  Save2DSignal=2-D array (concatenate along first dimension)
  M10 : ToWorkspace  VariableName=w_fdb_B  SampleTime=-1
      settings: Decimation=3  Save2DSignal=2-D array (concatenate along first dimension)
  M5 : ToWorkspace  VariableName=M_el_B  SampleTime=-1
      settings: Decimation=3  Save2DSignal=2-D array (concatenate along first dimension)
  M9 : ToWorkspace  VariableName=I_mr_B  SampleTime=-1
      settings: Decimation=3  Save2DSignal=2-D array (concatenate along first dimension)
  wires:
  Demux/4 -> M10/1
  Data/1 -> Demux/1
  Demux/1 -> M1/1
  Demux/2 -> M9/1
  Demux/3 -> M5/1

== system dq_model/motor2/Transformacije ==
  kot : Inport
  Udq : Inport  Port=2
  Inverzni Clarke : Subsystem
  Inverzni Park : Subsystem
  U123 : Outport
  wires:
  Inverzni Clarke/1(U_123) -> U123/1
  kot/1 -> Inverzni Park/1(kot)
  Inverzni Park/1(U_ab) -> Inverzni Clarke/1(U_ab)
  Udq/1 -> Inverzni Park/2(U_dq)

== system dq_model/Tehnika A/Regulacija navora/Limita q toka ==
  Iddej : Inport
  wmr : Inport  Port=2
  Iq* : Inport  Port=3
  MinMax : MinMax  Inputs=2
  Subsystem : Subsystem
  napetostna limita : Subsystem
  tokovna : Subsystem
  Iqmaxlim : Outport
  Iq*_lim : Outport  Port=2
  wires:
  wmr/1 -> napetostna limita/2(w)
  Iddej/1 -> napetostna limita/1(Iddej), tokovna/1(Id)
  MinMax/1 -> Subsystem/1(High), Iqmaxlim/1
  Iq*/1 -> Subsystem/2(U)
  Subsystem/1(Uq_lim) -> Iq*_lim/1
  napetostna limita/1(high) -> MinMax/1
  tokovna/1(high) -> MinMax/2

== system dq_model/Tehnika A/Tok regulator/Dregulator ==
  Id* : Inport
  Iddej : Inport  Port=2
  1/Ti : Gain  Gain=Ki_tok  SaturateOnIntegerOverflow=on  OutDataTypeStr=Inherit: Same as input  ParamDataTypeStr=Inherit: Same as input
  Abs : Abs  ZeroCross=off
  Add2 : Sum  Inputs=+-
  Compare To Zero : simulink/Logic and Bit Operations/Compare To Zero  relop=<=  OutDataTypeStr=boolean  ZeroCross=off
  Integrator : Integrator
  Kp : Gain  Gain=Kp_tok  SaturateOnIntegerOverflow=on  OutDataTypeStr=Inherit: Same as input  ParamDataTypeStr=Inherit: Same as input
  Product : Product
  Saturation : Saturate  UpperLimit=0.990  LowerLimit=-0.99  ZeroCross=off
  Scope : Scope  NumInputPorts=2
      settings: TimeRange=auto  MaxDataPoints=5000  SaveToWorkspace=off  SaveName=ScopeData6  YMin=-50.22005~-5  YMax=50.34382~5  SampleTime=-1
  Sum1 : Sum  Inputs=|+-
  Sum2 : Sum  Inputs=|++
  Ud*(-1:1) : Outport
  wires:
  Sum1/1 -> Product/1, Kp/1
  Add2/1 -> Abs/1
  Abs/1 -> Compare To Zero/1
  Iddej/1 -> Scope/2, Sum1/2
  1/Ti/1 -> Integrator/1
  Product/1 -> 1/Ti/1
  Kp/1 -> Sum2/1
  Compare To Zero/1 -> Product/2
  Sum2/1 -> Add2/1, Saturation/1
  Integrator/1 -> Sum2/2
  Id*/1 -> Scope/1, Sum1/1
  Saturation/1 -> Add2/2, Ud*(-1:1)/1

== system dq_model/Tehnika A/Tok regulator/Limita Uq ==
  Ud : Inport
  Uq : Inport  Port=2
  Abs : Abs  ZeroCross=off
  Add : Sum  Inputs=+-
  Constant1 : Constant
  Product3 : Product
  Scope : Scope
      settings: TimeRange=auto  MaxDataPoints=5000  SaveToWorkspace=off  SaveName=ScopeData3  YMin=0.0337  YMax=1.10737  SampleTime=-1
  Sqrt : Sqrt  SaturateOnIntegerOverflow=on
  Subsystem : Subsystem
  Uq_lim : Outport
  wires:
  Ud/1 -> Product3/1, Product3/2
  Uq/1 -> Subsystem/2(U)
  Subsystem/1(Uq_lim) -> Uq_lim/1
  Constant1/1 -> Add/1
  Product3/1 -> Add/2
  Add/1 -> Sqrt/1
  Sqrt/1 -> Abs/1
  Abs/1 -> Subsystem/1(High), Scope/1

== system dq_model/Tehnika A/Tok regulator/Qregulator ==
  Iqdej : Inport
  Iq* : Inport  Port=2
  Uqlim : Inport  Port=3
  1/Ti1 : Gain  Gain=Ki_tok  SaturateOnIntegerOverflow=on  OutDataTypeStr=Inherit: Same as input  ParamDataTypeStr=Inherit: Same as input
  Abs1 : Abs  ZeroCross=off
  Add1 : Sum  Inputs=+-
  Compare To Zero1 : simulink/Logic and Bit Operations/Compare To Zero  relop=<=  OutDataTypeStr=boolean  ZeroCross=off
  Integrator1 : Integrator
  Kp1 : Gain  Gain=Kp_tok  SaturateOnIntegerOverflow=on  OutDataTypeStr=Inherit: Same as input  ParamDataTypeStr=Inherit: Same as input
  Product1 : Product
  Scope : Scope  NumInputPorts=2
      settings: TimeRange=auto  MaxDataPoints=5000  SaveToWorkspace=off  SaveName=ScopeData2  YMin=-36.38891~-5  YMax=48.6611~5  SampleTime=-1
  Scope1 : Scope  NumInputPorts=2
      settings: TimeRange=auto  MaxDataPoints=5000  SaveToWorkspace=off  SaveName=ScopeData4  YMin=-0.125~-5  YMax=1.125~5  SampleTime=-1
  Sum3 : Sum  Inputs=|+-
  Sum4 : Sum  Inputs=|++
  Uq*(-1:1) : Outport
  wires:
  Iq*/1 -> Sum3/1, Scope/1
  Kp1/1 -> Sum4/1
  Integrator1/1 -> Sum4/2
  Sum3/1 -> Kp1/1, Product1/1
  Add1/1 -> Abs1/1
  Compare To Zero1/1 -> Scope1/1, Product1/2
  Product1/1 -> 1/Ti1/1
  1/Ti1/1 -> Integrator1/1
  Abs1/1 -> Compare To Zero1/1
  Iqdej/1 -> Sum3/2, Scope/2
  Uqlim/1 -> Add1/2
  Sum4/1 -> Uq*(-1:1)/1, Add1/1

== system dq_model/Tehnika B/Regulacija navora/Limita q toka ==
  Iddej : Inport
  wmr : Inport  Port=2
  Iq* : Inport  Port=3
  MinMax : MinMax  Inputs=2
  Scope : Scope  NumInputPorts=2
      settings: TimeRange=auto  MaxDataPoints=5000  SaveToWorkspace=off  SaveName=ScopeData4  YMin=28.79147~-5  YMax=41.42724~5  SampleTime=-1
  Subsystem : Subsystem
  napetostna limita : Subsystem
  tokovna : Subsystem
  Iqmaxlim : Outport
  Iq*_lim : Outport  Port=2
  wires:
  tokovna/1(high) -> MinMax/2
  napetostna limita/1(high) -> MinMax/1
  Subsystem/1(Uq_lim) -> Iq*_lim/1
  Iq*/1 -> Subsystem/2(U)
  MinMax/1 -> Subsystem/1(High), Iqmaxlim/1
  Iddej/1 -> tokovna/1(Id), napetostna limita/1(Iddej)
  wmr/1 -> napetostna limita/2(w)

== system dq_model/Tehnika B/TechniqueB1/Const c ==
  Id : Inport
  6.1-1 : TransferFcn  Numerator=[-Tr*Lm^2/Lr 0]  Denominator=[Tr 1]
  6.1-2 : TransferFcn  Denominator=[0.25 1]
  c : Outport
  wires:
  Id/1 -> 6.1-1/1
  6.1-1/1 -> 6.1-2/1
  6.1-2/1 -> c/1

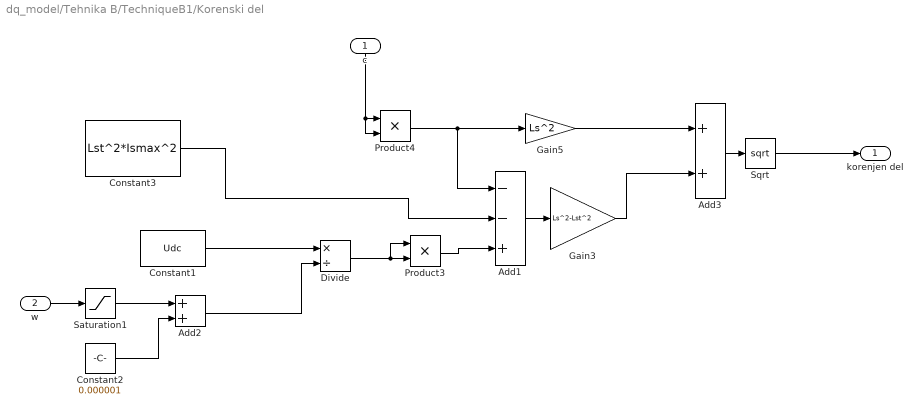
== system dq_model/Tehnika B/TechniqueB1/Korenski del ==
  c : Inport
  w : Inport  Port=2
  Add1 : Sum  Inputs=--+
  Add2 : Sum
  Add3 : Sum
  Constant1 : Constant  Value=Udc
  Constant2 : Constant  Value=0.000001
  Constant3 : Constant  Value=Lst^2*Ismax^2
  Divide : Product  Inputs=*/
  Gain3 : Gain  Gain=Ls^2-Lst^2
  Gain5 : Gain  Gain=Ls^2
  Product3 : Product
  Product4 : Product
  Saturation1 : Saturate  UpperLimit=wb_upper_limit_field_weaking  LowerLimit=-wb_upper_limit_field_weaking
  Sqrt : Sqrt  SaturateOnIntegerOverflow=on
  korenjen del : Outport
  wires:
  c/1 -> Product4/2, Product4/1
  Product4/1 -> Add1/1, Gain5/1
  Saturation1/1 -> Add2/1
  Constant1/1 -> Divide/1
  Constant2/1 -> Add2/2
  Add1/1 -> Gain3/1
  Add2/1 -> Divide/2
  w/1 -> Saturation1/1
  Divide/1 -> Product3/1, Product3/2
  Product3/1 -> Add1/3
  Sqrt/1 -> korenjen del/1
  Add3/1 -> Sqrt/1
  Gain5/1 -> Add3/1
  Gain3/1 -> Add3/2
  Constant3/1 -> Add1/2

== system dq_model/Tehnika B/Tok regulator/Dregulator ==
  Id* : Inport
  Iddej : Inport  Port=2
  1/Ti : Gain  Gain=Ki_tok  SaturateOnIntegerOverflow=on  OutDataTypeStr=Inherit: Same as input  ParamDataTypeStr=Inherit: Same as input
  Abs : Abs  ZeroCross=off
  Add2 : Sum  Inputs=+-
  Compare To Zero : simulink/Logic and Bit Operations/Compare To Zero  relop=<=  OutDataTypeStr=boolean  ZeroCross=off
  Integrator : Integrator
  Kp : Gain  Gain=Kp_tok  SaturateOnIntegerOverflow=on  OutDataTypeStr=Inherit: Same as input  ParamDataTypeStr=Inherit: Same as input
  Product : Product
  Saturation : Saturate  UpperLimit=0.990  LowerLimit=-0.99  ZeroCross=off
  Scope : Scope  NumInputPorts=2
      settings: TimeRange=auto  MaxDataPoints=5000  SaveToWorkspace=off  SaveName=ScopeData6  YMin=-50.22005~-5  YMax=50.34382~5  SampleTime=-1
  Sum1 : Sum  Inputs=|+-
  Sum2 : Sum  Inputs=|++
  Ud*(-1:1) : Outport
  wires:
  Saturation/1 -> Ud*(-1:1)/1, Add2/2
  Id*/1 -> Sum1/1, Scope/1
  Integrator/1 -> Sum2/2
  Sum2/1 -> Saturation/1, Add2/1
  Compare To Zero/1 -> Product/2
  Kp/1 -> Sum2/1
  Product/1 -> 1/Ti/1
  1/Ti/1 -> Integrator/1
  Iddej/1 -> Sum1/2, Scope/2
  Abs/1 -> Compare To Zero/1
  Add2/1 -> Abs/1
  Sum1/1 -> Kp/1, Product/1

== system dq_model/Tehnika B/Tok regulator/Limita Uq ==
  Ud : Inport
  Uq : Inport  Port=2
  Abs : Abs  ZeroCross=off
  Add : Sum  Inputs=+-
  Constant1 : Constant
  Product3 : Product
  Scope : Scope
      settings: TimeRange=auto  MaxDataPoints=5000  SaveToWorkspace=off  SaveName=ScopeData3  YMin=0.0337  YMax=1.10737  SampleTime=-1
  Sqrt : Sqrt  SaturateOnIntegerOverflow=on
  Subsystem : Subsystem
  Uq_lim : Outport
  wires:
  Product3/1 -> Add/2
  Constant1/1 -> Add/1
  Ud/1 -> Product3/2, Product3/1
  Add/1 -> Abs/1
  Abs/1 -> Sqrt/1
  Sqrt/1 -> Subsystem/1(High), Scope/1
  Uq/1 -> Subsystem/2(U)
  Subsystem/1(Uq_lim) -> Uq_lim/1

== system dq_model/Tehnika B/Tok regulator/Qregulator ==
  Iqdej : Inport
  Iq* : Inport  Port=2
  Uqlim : Inport  Port=3
  1/Ti1 : Gain  Gain=Ki_tok  SaturateOnIntegerOverflow=on  OutDataTypeStr=Inherit: Same as input  ParamDataTypeStr=Inherit: Same as input
  Abs1 : Abs  ZeroCross=off
  Add1 : Sum  Inputs=+-
  Compare To Zero1 : simulink/Logic and Bit Operations/Compare To Zero  relop=<=  OutDataTypeStr=boolean  ZeroCross=off
  Integrator1 : Integrator
  Kp1 : Gain  Gain=Kp_tok  SaturateOnIntegerOverflow=on  OutDataTypeStr=Inherit: Same as input  ParamDataTypeStr=Inherit: Same as input
  Product1 : Product
  Scope : Scope  NumInputPorts=2
      settings: TimeRange=auto  MaxDataPoints=5000  SaveToWorkspace=off  SaveName=ScopeData2  YMin=-36.38891~-5  YMax=48.6611~5  SampleTime=-1
  Scope1 : Scope  NumInputPorts=2
      settings: TimeRange=auto  MaxDataPoints=5000  SaveToWorkspace=off  SaveName=ScopeData4  YMin=-0.125~-5  YMax=1.125~5  SampleTime=-1
  Sum3 : Sum  Inputs=|+-
  Sum4 : Sum  Inputs=|++
  Uq*(-1:1) : Outport
  wires:
  Sum4/1 -> Add1/1, Uq*(-1:1)/1
  Uqlim/1 -> Add1/2
  Iqdej/1 -> Scope/2, Sum3/2
  Abs1/1 -> Compare To Zero1/1
  1/Ti1/1 -> Integrator1/1
  Product1/1 -> 1/Ti1/1
  Compare To Zero1/1 -> Product1/2, Scope1/1
  Add1/1 -> Abs1/1
  Sum3/1 -> Product1/1, Kp1/1
  Integrator1/1 -> Sum4/2
  Kp1/1 -> Sum4/1
  Iq*/1 -> Scope/1, Sum3/1

== system dq_model/Tehnika s/Regulacija navora/Limita q toka ==
  Iddej : Inport
  wmr : Inport  Port=2
  Iq* : Inport  Port=3
  Gain : Gain  Gain=-1
  MinMax : MinMax  Inputs=2
  Saturation napetost : simulink/Discontinuities/Saturation Dynamic  OutMin=[]  OutMax=[]  OutDataTypeStr=Inherit: Same as second input  OutDataType=fixdt(1, 16)  OutScaling=2^-10  DoSatur=off
  Scope : Scope  NumInputPorts=2
      settings: TimeRange=auto  MaxDataPoints=5000  SaveToWorkspace=off  SaveName=ScopeData4  YMin=28.79147~-5  YMax=41.42724~5  SampleTime=-1
  napetostna limita : Subsystem
  tokovna : Subsystem
  Iqmaxlim : Outport
  Iq*_lim : Outport  Port=2
  wires:
  tokovna/1(high) -> MinMax/2
  napetostna limita/1(high) -> MinMax/1
  Gain/1 -> Saturation napetost/3
  Saturation napetost/1 -> Iq*_lim/1
  Iq*/1 -> Saturation napetost/2
  MinMax/1 -> Gain/1, Iqmaxlim/1, Saturation napetost/1
  Iddej/1 -> tokovna/1(Id), napetostna limita/1(Iddej)
  wmr/1 -> napetostna limita/2(w)

== system dq_model/Tehnika s/Tok regulator/Dregulator ==
  Id* : Inport
  Iddej : Inport  Port=2
  1/Ti : Gain  Gain=Ki_tok  SaturateOnIntegerOverflow=on  OutDataTypeStr=Inherit: Same as input  ParamDataTypeStr=Inherit: Same as input
  Abs : Abs  ZeroCross=off
  Add2 : Sum  Inputs=+-
  Compare To Zero : simulink/Logic and Bit Operations/Compare To Zero  relop=<=  OutDataTypeStr=boolean  ZeroCross=off
  Integrator : Integrator
  Kp : Gain  Gain=Kp_tok  SaturateOnIntegerOverflow=on  OutDataTypeStr=Inherit: Same as input  ParamDataTypeStr=Inherit: Same as input
  Product : Product
  Saturation : Saturate  UpperLimit=0.990  LowerLimit=-0.99  ZeroCross=off
  Scope : Scope  NumInputPorts=2
      settings: TimeRange=auto  MaxDataPoints=5000  SaveToWorkspace=off  SaveName=ScopeData6  YMin=-50.22005~-5  YMax=50.34382~5  SampleTime=-1
  Sum1 : Sum  Inputs=|+-
  Sum2 : Sum  Inputs=|++
  Ud*(-1:1) : Outport
  wires:
  Saturation/1 -> Ud*(-1:1)/1, Add2/2
  Id*/1 -> Sum1/1, Scope/1
  Integrator/1 -> Sum2/2
  Sum2/1 -> Saturation/1, Add2/1
  Compare To Zero/1 -> Product/2
  Kp/1 -> Sum2/1
  Product/1 -> 1/Ti/1
  1/Ti/1 -> Integrator/1
  Iddej/1 -> Sum1/2, Scope/2
  Abs/1 -> Compare To Zero/1
  Add2/1 -> Abs/1
  Sum1/1 -> Kp/1, Product/1

== system dq_model/Tehnika s/Tok regulator/Limita Uq ==
  Ud : Inport
  Uq : Inport  Port=2
  Abs : Abs  ZeroCross=off
  Add : Sum  Inputs=+-
  Constant1 : Constant
  Product3 : Product
  Scope : Scope
      settings: TimeRange=auto  MaxDataPoints=5000  SaveToWorkspace=off  SaveName=ScopeData3  YMin=0.0337  YMax=1.10737  SampleTime=-1
  Sqrt : Sqrt  SaturateOnIntegerOverflow=on
  Subsystem : Subsystem
  Uq_lim : Outport
  wires:
  Abs/1 -> Subsystem/1(High), Scope/1
  Sqrt/1 -> Abs/1
  Add/1 -> Sqrt/1
  Product3/1 -> Add/2
  Constant1/1 -> Add/1
  Subsystem/1(Uq_lim) -> Uq_lim/1
  Uq/1 -> Subsystem/2(U)
  Ud/1 -> Product3/2, Product3/1

== system dq_model/Tehnika s/Tok regulator/Qregulator ==
  Iqdej : Inport
  Iq* : Inport  Port=2
  Uqlim : Inport  Port=3
  1/Ti1 : Gain  Gain=100  SaturateOnIntegerOverflow=on  OutDataTypeStr=Inherit: Same as input  ParamDataTypeStr=Inherit: Same as input
  Abs1 : Abs  ZeroCross=off
  Add1 : Sum  Inputs=+-
  Compare To Zero1 : simulink/Logic and Bit Operations/Compare To Zero  relop=<=  OutDataTypeStr=boolean  ZeroCross=off
  Integrator1 : Integrator
  Kp1 : Gain  Gain=0.05  SaturateOnIntegerOverflow=on  OutDataTypeStr=Inherit: Same as input  ParamDataTypeStr=Inherit: Same as input
  Product1 : Product
  Scope : Scope  NumInputPorts=2
      settings: TimeRange=auto  MaxDataPoints=5000  SaveToWorkspace=off  SaveName=ScopeData2  YMin=-36.38891~-5  YMax=48.6611~5  SampleTime=-1
  Scope1 : Scope  NumInputPorts=2
      settings: TimeRange=auto  MaxDataPoints=5000  SaveToWorkspace=off  SaveName=ScopeData4  YMin=-0.125~-5  YMax=1.125~5  SampleTime=-1
  Sum3 : Sum  Inputs=|+-
  Sum4 : Sum  Inputs=|++
  Uq*(-1:1) : Outport
  wires:
  Sum4/1 -> Add1/1, Uq*(-1:1)/1
  Uqlim/1 -> Add1/2
  Iqdej/1 -> Scope/2, Sum3/2
  Abs1/1 -> Compare To Zero1/1
  1/Ti1/1 -> Integrator1/1
  Product1/1 -> 1/Ti1/1
  Compare To Zero1/1 -> Product1/2, Scope1/1
  Add1/1 -> Abs1/1
  Sum3/1 -> Product1/1, Kp1/1
  Integrator1/1 -> Sum4/2
  Kp1/1 -> Sum4/1
  Iq*/1 -> Scope/1, Sum3/1

== system dq_model/motor/Asinhronski stroj1/Clarke ==
  U_123 : Inport
  ABC_ab1 : Subsystem
  Demux : Demux  Outputs=3
  Mux : Mux  Inputs=2
  U_ab : Outport
  wires:
  Mux/1 -> U_ab/1
  ABC_ab1/2(beta) -> Mux/2
  ABC_ab1/1(alfa) -> Mux/1
  Demux/3 -> ABC_ab1/3(C)
  Demux/2 -> ABC_ab1/2(B)
  Demux/1 -> ABC_ab1/1(A)
  U_123/1 -> Demux/1

== system dq_model/motor/Asinhronski stroj1/Inverzni Clarke ==
  I_ab : Inport
  Demux : Demux  Outputs=2
  Mux : Mux  Inputs=3
  ab_ABC : Subsystem
  I_123 : Outport
  wires:
  ab_ABC/3(C) -> Mux/3
  ab_ABC/2(B) -> Mux/2
  ab_ABC/1(A) -> Mux/1
  Demux/2 -> ab_ABC/2(beta)
  Demux/1 -> ab_ABC/1(alfa)
  I_ab/1 -> Demux/1
  Mux/1 -> I_123/1

== system dq_model/motor/Asinhronski stroj1/Inverzni Park ==
  I_dq : Inport
  kot : Inport  Port=2
  Demux : Demux  Outputs=2
  Mux : Mux  Inputs=2
  "Sum1 " : Sum  Inputs=+-  SaturateOnIntegerOverflow=on  InputSameDT=on  OutDataTypeStr=Inherit: Same as first input
  Sum2 : Sum  SaturateOnIntegerOverflow=on  InputSameDT=on  OutDataTypeStr=Inherit: Same as first input
  cos : Fcn  Expr=cos(u)
  sin : Fcn  Expr=sin(u)
  x_d*cos : Product  SaturateOnIntegerOverflow=on  RndMeth=Zero  InputSameDT=on  OutDataTypeStr=Inherit: Same as first input
  x_d*sin : Product  SaturateOnIntegerOverflow=on  RndMeth=Zero  InputSameDT=on  OutDataTypeStr=Inherit: Same as first input
  x_q*cos : Product  SaturateOnIntegerOverflow=on  RndMeth=Zero  InputSameDT=on  OutDataTypeStr=Inherit: Same as first input
  "x_q*sin " : Product  SaturateOnIntegerOverflow=on  RndMeth=Zero  InputSameDT=on  OutDataTypeStr=Inherit: Same as first input
  I_ab : Outport
  wires:
  Mux/1 -> I_ab/1
  I_dq/1 -> Demux/1
  Demux/1 -> x_d*sin/1, x_d*cos/1
  Demux/2 -> "x_q*sin "/1, x_q*cos/1
  cos/1 -> x_q*cos/2, x_d*cos/2
  sin/1 -> "x_q*sin "/2, x_d*sin/2
  x_d*cos/1 -> "Sum1 "/1
  "x_q*sin "/1 -> "Sum1 "/2
  x_q*cos/1 -> Sum2/2
  x_d*sin/1 -> Sum2/1
  "Sum1 "/1 -> Mux/1
  Sum2/1 -> Mux/2
  kot/1 -> cos/1, sin/1

== system dq_model/motor/Asinhronski stroj1/Mehanika ==
  M_br : Inport
  M_el : Inport  Port=2
  Sum : Sum  Inputs=+-
  eq 2.19 : Subsystem
  wr : Outport
  wires:
  M_br/1 -> Sum/2
  Sum/1 -> eq 2.19/1(M)
  M_el/1 -> Sum/1
  eq 2.19/1(wr) -> wr/1

== system dq_model/motor/Asinhronski stroj1/Park ==
  U_ab : Inport
  kot : Inport  Port=2
  Demux : Demux  Outputs=2
  Mux : Mux  Inputs=2
  "Sum1 " : Sum  SaturateOnIntegerOverflow=on  InputSameDT=on  OutDataTypeStr=Inherit: Same as first input
  Sum2 : Sum  Inputs=-+  SaturateOnIntegerOverflow=on  InputSameDT=on  OutDataTypeStr=Inherit: Same as first input
  cos : Fcn  Expr=cos(u)
  sin : Fcn  Expr=sin(u)
  x_a*cos : Product  SaturateOnIntegerOverflow=on  RndMeth=Zero  InputSameDT=on  OutDataTypeStr=Inherit: Same as first input
  x_a*sin : Product  SaturateOnIntegerOverflow=on  RndMeth=Zero  InputSameDT=on  OutDataTypeStr=Inherit: Same as first input
  x_b*cos : Product  SaturateOnIntegerOverflow=on  RndMeth=Zero  InputSameDT=on  OutDataTypeStr=Inherit: Same as first input
  "x_b*sin " : Product  SaturateOnIntegerOverflow=on  RndMeth=Zero  InputSameDT=on  OutDataTypeStr=Inherit: Same as first input
  U_dq : Outport
  wires:
  Mux/1 -> U_dq/1
  U_ab/1 -> Demux/1
  Demux/1 -> x_a*sin/1, x_a*cos/1
  Demux/2 -> "x_b*sin "/1, x_b*cos/1
  cos/1 -> x_b*cos/2, x_a*cos/2
  sin/1 -> "x_b*sin "/2, x_a*sin/2
  x_a*cos/1 -> "Sum1 "/1
  "x_b*sin "/1 -> "Sum1 "/2
  x_b*cos/1 -> Sum2/2
  x_a*sin/1 -> Sum2/1
  "Sum1 "/1 -> Mux/1
  Sum2/1 -> Mux/2
  kot/1 -> cos/1, sin/1

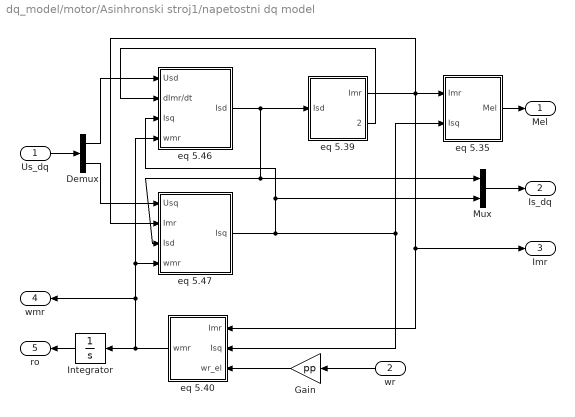
== system dq_model/motor/Asinhronski stroj1/napetostni dq model ==
  Us_dq : Inport
  wr : Inport  Port=2
  Demux : Demux  Outputs=2
  Gain : Gain  Gain=pp
  Integrator : Integrator
  Mux : Mux  Inputs=2
  eq 5.35 : Subsystem
  eq 5.39 : Subsystem
  eq 5.40 : Subsystem
  eq 5.46 : Subsystem
  eq 5.47 : Subsystem
  Mel : Outport
  Is_dq : Outport  Port=2
  Imr : Outport  Port=3
  wmr : Outport  Port=4
  ro : Outport  Port=5
  wires:
  Gain/1 -> eq 5.40/3(wr_el)
  Mux/1 -> Is_dq/1
  Demux/2 -> eq 5.47/1(Usq)
  Demux/1 -> eq 5.46/1(Usd)
  Us_dq/1 -> Demux/1
  wr/1 -> Gain/1
  Integrator/1 -> ro/1
  eq 5.35/1(Mel) -> Mel/1
  eq 5.40/1(wmr) -> Integrator/1, wmr/1, eq 5.46/4(wmr), eq 5.47/4(wmr)
  eq 5.47/1(Isq) -> Mux/2, eq 5.46/3(Isq), eq 5.40/2(Isq), eq 5.35/2(Isq)
  eq 5.39/1(Imr) -> eq 5.47/2(Imr), Imr/1, eq 5.40/1(Imr), eq 5.35/1(Imr)
  eq 5.39/2(dImr/dt) -> eq 5.46/2(dImr/dt)
  eq 5.46/1(Isd) -> Mux/1, eq 5.47/3(Isd), eq 5.39/1(Isd)

== system dq_model/motor/Transformacije/Inverzni Clarke ==
  U_ab : Inport
  Demux : Demux  Outputs=2
  Mux : Mux  Inputs=3
  ab_ABC : Subsystem
  U_123 : Outport
  wires:
  ab_ABC/3(C) -> Mux/3
  ab_ABC/2(B) -> Mux/2
  ab_ABC/1(A) -> Mux/1
  Demux/2 -> ab_ABC/2(beta)
  Demux/1 -> ab_ABC/1(alfa)
  U_ab/1 -> Demux/1
  Mux/1 -> U_123/1
